simulink model "speedgoat_test_SN5659_R2021b"  (R2021b)
settings: Solver=FixedStepDiscrete  StartTime=0.0  StopTime=inf  RelTol=1e-3
PreLoadFcn:
  | Ts_IO107 = 0.001;
  | Ts_IO107 = 0.001;
  | Ts_IO133 = 0.001
  | 
  | Ts_IO204 = 0.001;
  | 
  | 
  | Ts_IO503 = 0.01;
  | 
  | ts_IO612 = 1e-3;
  | Ts_IO682 = 0.005;
  | Ts_IO941 = 0.01;
InitFcn:
  | Ts_IO107 = 0.001;
  | Ts_IO107 = 0.001;
  | Ts_IO133 = 0.001
  | 
  | Ts_IO204 = 0.001;
  | 
  | 
  | Ts_IO503 = 0.01;
  | 
  | ts_IO612 = 1e-3;
  | Ts_IO682 = 0.005;
  | Ts_IO941 = 0.01;
StopFcn:
  | if isfile(['sdi_view_',bdroot,'.mldatx'])
  |  Simulink.sdi.clearPreferences();
  |  Simulink.sdi.view();
  |  pause(3);
  |  Simulink.sdi.loadView(['sdi_view_',bdroot,]);
  | end
undefined symbols (not defined in the file): C, IO682, standard
libraries: speedgoatlib_IO682 x161, simulink x49, slrealtimeseriallib x16, canmsglib x12, speedgoatlib_serial x9, speedgoatlib_IO612 x9, speedgoatlib_IO133 x5, speedgoatlib_IO107 x4, speedgoatlib_IO204 x3, speedgoatlib_IO421 x3, speedgoatlib_PIL x1
(part 4 of 4)

== system speedgoat_test_SN5659_R2021b/IO682/Encode Channel 9/Prepare RAW value ==
  note: The scale factor is
      | defined by the label
      | for this message.
  note: Manually construct the ARINC word.
      | This sample constructs a BNR format
      | word, but the data part could be
      | constructed from multiple data pieces
      | and discrete bits if the label requires it.
  note: Data
  note: The output has to be cast to a double
      | for input to the ARINC Encode block.
  note: The data could be constructed direcly as an integer if needed.
  note: Octal 103 = decimal 67 = hex 43
  In1 : Inport
  'shift' the double value 27 bits left : Constant  Value=2^28  OutDataTypeStr=double
  Bitwise Operator : simulink/Logic and Bit Operations/Bitwise Operator  logicop=OR  UseBitMask=off  NumInputPorts=4  BitMask=bin2dec('11011001')  BitMaskRealWorld=Stored Integer
  Data Type Conversion : DataTypeConversion  OutDataTypeStr=uint32
  Data Type Conversion1 : DataTypeConversion  OutDataTypeStr=double
  Display : Display
      settings: Format=hex (Stored Integer)
  Divide : Product  Inputs=*/
  Label : Constant  Value=base2dec( '103', 8 )  OutDataTypeStr=uint32
  "Mask " : simulink/Logic and Bit Operations/Bitwise Operator  logicop=AND  UseBitMask=on  BitMask=hex2dec('1ffffc00')  BitMaskRealWorld=Stored Integer
  Multiply : Product  Inputs=**
  SDI : Constant  Value=2  OutDataTypeStr=uint32
  SSM : Constant  Value=3  OutDataTypeStr=uint32
  Scale : Constant  Value=1024  OutDataTypeStr=double
  Shift to SDI slot : ArithShift  BitShiftNumber=-8
  Shift to SSM slot : ArithShift  BitShiftNumber=-29
  Out1 : Outport
  wires:
  In1/1 -> Divide/1
  Scale/1 -> Divide/2
  'shift' the double value 27 bits left/1 -> Multiply/2
  Divide/1 -> Multiply/1
  Multiply/1 -> Data Type Conversion/1
  Data Type Conversion/1 -> "Mask "/1
  "Mask "/1 -> Bitwise Operator/1
  SSM/1 -> Shift to SSM slot/1
  SDI/1 -> Shift to SDI slot/1
  Shift to SSM slot/1 -> Bitwise Operator/2
  Shift to SDI slot/1 -> Bitwise Operator/3
  Label/1 -> Bitwise Operator/4
  Bitwise Operator/1 -> Data Type Conversion1/1, Display/1
  Data Type Conversion1/1 -> Out1/1
